simulink model "EvitarObstaculo"  (R2020b)
settings: Solver=ode3  StartTime=0.0  StopTime=100.0  FixedStep=Ts  RelTol=1e-3
values from neighbouring files (symbols this model uses):
  obsx = 4    [Ejercicio1.m]    (also in Ejercicio2.m = 2.03)
  obsy = 0    [Ejercicio1.m]    (also in Ejercicio2.m = 1)
  refx = 9    [Ejercicio1.m]
  refy = 0    [Ejercicio1.m]
undefined symbols (not defined in the file or in its folder): DiscIntNeverNeededParam
libraries: fuzblock x1, simulink x1
settings Model: Creator=patri  LastModifiedBy=patri
settings DataIOCC: SaveOutput=off  ReturnWorkspaceOutputs=off

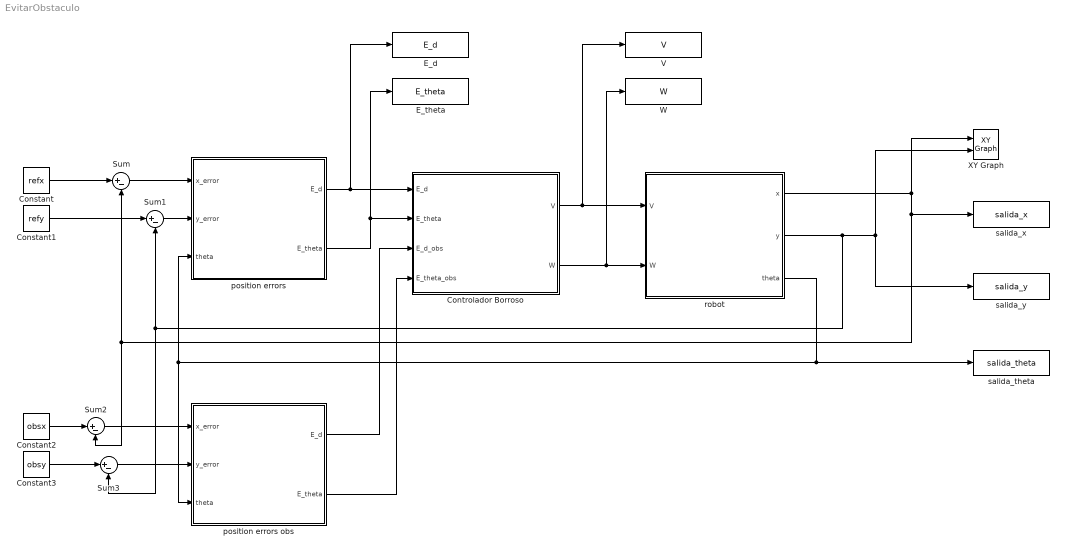
== system EvitarObstaculo ==
  Constant : Constant  Value=refx
  Constant1 : Constant  Value=refy
  Constant2 : Constant  Value=obsx
  Constant3 : Constant  Value=obsy
  Controlador Borroso : Subsystem
  E_d : ToWorkspace  VariableName=E_d  SaveFormat=Structure With Time  SampleTime=-1
  E_theta : ToWorkspace  VariableName=E_theta  SaveFormat=Structure With Time  SampleTime=-1
  Sum{,1..3} (4 alike) : Sum  Inputs=|+-
  V : ToWorkspace  VariableName=V  SaveFormat=Structure With Time  SampleTime=-1
  W : ToWorkspace  VariableName=W  SaveFormat=Structure With Time  SampleTime=-1
  XY Graph : simulink/Sinks/XY Graph  xmin=-10  xmax=10  ymin=-10  ymax=10  st=-1
  position errors : Subsystem
  position errors obs : Subsystem
  robot : Subsystem
  salida_theta : ToWorkspace  VariableName=salida_theta  SaveFormat=Structure With Time  SampleTime=-1
  salida_x : ToWorkspace  VariableName=salida_x  SaveFormat=Structure With Time  SampleTime=-1
  salida_y : ToWorkspace  VariableName=salida_y  SaveFormat=Structure With Time  SampleTime=-1
  wires:
  Sum1/1 -> position errors/2(y_error)
  position errors/2(E_theta) -> Controlador Borroso/2(E_theta), E_theta/1
  Controlador Borroso/1(V) -> robot/1(V), V/1
  robot/2(y) -> salida_y/1, XY Graph/2, Sum1/2, Sum3/2
  Controlador Borroso/2(W) -> robot/2(W), W/1
  Sum/1 -> position errors/1(x_error)
  position errors/1(E_d) -> Controlador Borroso/1(E_d), E_d/1
  robot/3(theta) -> salida_theta/1, position errors obs/3(theta), position errors/3(theta)
  Constant/1 -> Sum/1
  Constant1/1 -> Sum1/1
  Constant2/1 -> Sum2/1
  Constant3/1 -> Sum3/1
  robot/1(x) -> salida_x/1, Sum/2, Sum2/2, XY Graph/1
  Sum2/1 -> position errors obs/1(x_error)
  Sum3/1 -> position errors obs/2(y_error)
  position errors obs/1(E_d) -> Controlador Borroso/3(E_d_obs)
  position errors obs/2(E_theta) -> Controlador Borroso/4(E_theta_obs)

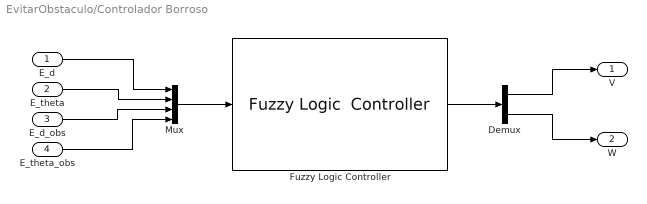
== system EvitarObstaculo/Controlador Borroso ==
  E_d : Inport
  E_theta : Inport  Port=2
  E_d_obs : Inport  Port=3
  E_theta_obs : Inport  Port=4
  Demux : Demux  Outputs=2
  Fuzzy Logic Controller : fuzblock/Fuzzy Logic  Controller  FIS='ControlBorroso.fis'  OutputSampleNumber=101  DataType=double  FuzzifiedInputs=off  RuleFiringStrengths=off  RuleOutputs=off  AggregatedOutputs=off  SimulateUsing=Interpreted execution  OutOfRangeInputValueMessage=warning  NoRuleFiredMessage=warning  EmptyOutputFuzzySetMessage=warning
  Mux : Mux
  V : Outport
  W : Outport  Port=2
  wires:
  Mux/1 -> Fuzzy Logic Controller/1
  E_theta/1 -> Mux/2
  Demux/1 -> V/1
  Fuzzy Logic Controller/1 -> Demux/1
  E_d/1 -> Mux/1
  Demux/2 -> W/1
  E_d_obs/1 -> Mux/3
  E_theta_obs/1 -> Mux/4

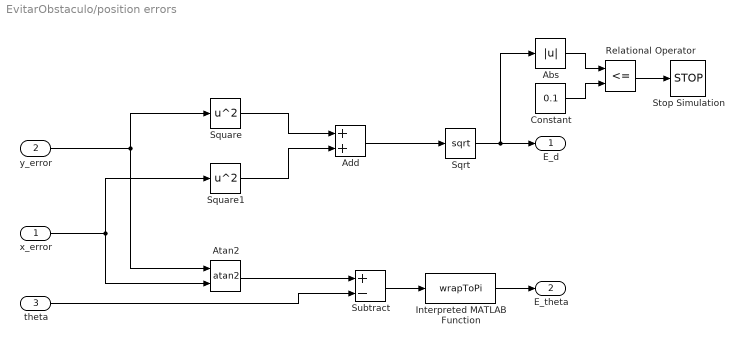
== system EvitarObstaculo/position errors ==
  x_error : Inport
  y_error : Inport  Port=2
  theta : Inport  Port=3
  Abs : Abs
  Add : Sum
  Atan2 : Trigonometry  Operator=atan2
  Constant : Constant  Value=0.1
  Interpreted MATLAB Function : MATLABFcn  MATLABFcn=wrapToPi
  Relational Operator : RelationalOperator  Operator=<=  OutDataTypeStr=boolean  RndMeth=Simplest
  Sqrt : Sqrt  SaturateOnIntegerOverflow=on
  Square : Math  Operator=square  SignedPower=on  SaturateOnIntegerOverflow=on
  Square1 : Math  Operator=square  SignedPower=on  SaturateOnIntegerOverflow=on
  Stop Simulation : Stop
  Subtract : Sum  Inputs=+-
  E_d : Outport  VectorParamsAs1DForOutWhenUnconnected=off
  E_theta : Outport  Port=2  OutMin=[-pi]  OutMax=[pi]  VectorParamsAs1DForOutWhenUnconnected=off
  wires:
  Subtract/1 -> Interpreted MATLAB Function/1
  theta/1 -> Subtract/2
  Constant/1 -> Relational Operator/2
  Interpreted MATLAB Function/1 -> E_theta/1
  Add/1 -> Sqrt/1
  Atan2/1 -> Subtract/1
  Abs/1 -> Relational Operator/1
  Sqrt/1 -> Abs/1, E_d/1
  Relational Operator/1 -> Stop Simulation/1
  Square1/1 -> Add/2
  y_error/1 -> Atan2/1, Square/1
  x_error/1 -> Atan2/2, Square1/1
  Square/1 -> Add/1

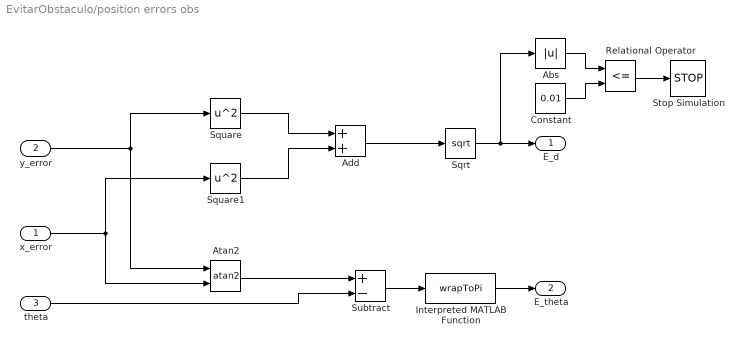
== system EvitarObstaculo/position errors obs ==
  x_error : Inport
  y_error : Inport  Port=2
  theta : Inport  Port=3
  Abs : Abs
  Add : Sum
  Atan2 : Trigonometry  Operator=atan2
  Constant : Constant  Value=0.01
  Interpreted MATLAB Function : MATLABFcn  MATLABFcn=wrapToPi
  Relational Operator : RelationalOperator  Operator=<=  OutDataTypeStr=boolean  RndMeth=Simplest
  Sqrt : Sqrt  SaturateOnIntegerOverflow=on
  Square : Math  Operator=square  SignedPower=on  SaturateOnIntegerOverflow=on
  Square1 : Math  Operator=square  SignedPower=on  SaturateOnIntegerOverflow=on
  Stop Simulation : Stop
  Subtract : Sum  Inputs=+-
  E_d : Outport  VectorParamsAs1DForOutWhenUnconnected=off
  E_theta : Outport  Port=2  OutMin=[-pi]  OutMax=[pi]  VectorParamsAs1DForOutWhenUnconnected=off
  wires:
  Sqrt/1 -> Abs/1, E_d/1
  y_error/1 -> Atan2/1, Square/1
  Interpreted MATLAB Function/1 -> E_theta/1
  Square/1 -> Add/1
  Constant/1 -> Relational Operator/2
  Square1/1 -> Add/2
  Subtract/1 -> Interpreted MATLAB Function/1
  Relational Operator/1 -> Stop Simulation/1
  theta/1 -> Subtract/2
  Atan2/1 -> Subtract/1
  x_error/1 -> Atan2/2, Square1/1
  Add/1 -> Sqrt/1
  Abs/1 -> Relational Operator/1

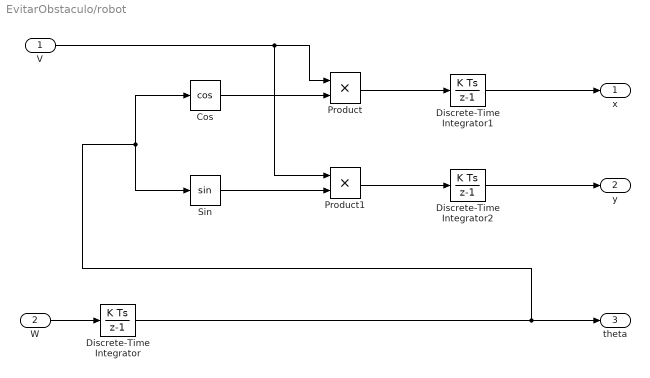
== system EvitarObstaculo/robot ==
  V : Inport
  W : Inport  Port=2
  Cos : Trigonometry  Operator=cos
  Discrete-Time Integrator : DiscreteIntegrator  SampleTime=-1  ICPrevOutput=DiscIntNeverNeededParam  ICPrevScaledInput=DiscIntNeverNeededParam
  Discrete-Time Integrator1 : DiscreteIntegrator  SampleTime=-1  ICPrevOutput=DiscIntNeverNeededParam  ICPrevScaledInput=DiscIntNeverNeededParam
  Discrete-Time Integrator2 : DiscreteIntegrator  SampleTime=-1  ICPrevOutput=DiscIntNeverNeededParam  ICPrevScaledInput=DiscIntNeverNeededParam
  Product : Product
  Product1 : Product
  Sin : Trigonometry
  x : Outport  VectorParamsAs1DForOutWhenUnconnected=off
  y : Outport  Port=2  VectorParamsAs1DForOutWhenUnconnected=off
  theta : Outport  Port=3  VectorParamsAs1DForOutWhenUnconnected=off
  wires:
  Discrete-Time Integrator/1 -> Sin/1, Cos/1, theta/1
  W/1 -> Discrete-Time Integrator/1
  Cos/1 -> Product/2
  Sin/1 -> Product1/2
  Discrete-Time Integrator1/1 -> x/1
  Discrete-Time Integrator2/1 -> y/1
  Product/1 -> Discrete-Time Integrator1/1
  V/1 -> Product1/1, Product/1
  Product1/1 -> Discrete-Time Integrator2/1
